simulink model "Simulink_6DoF_RV"  (R2021b)
settings: Solver=ode4  StartTime=0.0  StopTime=T_run  FixedStep=0.01  RelTol=1e-3
values from neighbouring files (symbols this model uses):
  alpha = 5    [MAIN_6DoF_RV.m]    (also in Simulatore_script_gruppo6.m)
  beta = 10    [MAIN_6DoF_RV.m]    (also in Simulatore_script_gruppo6.m)
  control = 2    [MAIN_6DoF_RV.m]    (also in Simulatore_script_gruppo6.m)
  den_pos = [Tm_pos 1]    [MAIN_6DoF_RV.m]    (also in Simulatore_script_gruppo6.m)
  dt_Fx1_PH1 = (1+dtx_PH1_corr)*dt_Fx1_PH1id    (= 48.314973357)    [MAIN_6DoF_RV.m]    (also in Simulatore_script_gruppo6.m)
  Dt_var = 0.1    [MAIN_6DoF_RV.m]    (also in Simulatore_script_gruppo6.m)
  dtz_PH2_corr = 0.28    [MAIN_6DoF_RV.m]    (also in Simulatore_script_gruppo6.m)
  epsilon = 1e-3    (= 0.001)    [MAIN_6DoF_RV.m]    (also in Simulatore_script_gruppo6.m)
  epsilon_FA = 0.005    [MAIN_6DoF_RV.m]    (also in Simulatore_script_gruppo6.m)
  F_D = 1/2*rho*CD*A*vc^2    [MAIN_6DoF_RV.m]    (also in Simulatore_script_gruppo6.m)
  fa_control = 2    [MAIN_6DoF_RV.m]    (also in Simulatore_script_gruppo6.m)
  FJ2_r4 = -mc*(3*J2*mu*r_E^2)/2    (= -1.15338103268e+24)    [MAIN_6DoF_RV.m]    (also in Simulatore_script_gruppo6.m)
  Fx_PH1id = Tmax    (= 1)    [MAIN_6DoF_RV.m]    (also in Simulatore_script_gruppo6.m)
  Fz_PH2id = Tmax    (= 1)    [MAIN_6DoF_RV.m]    (also in Simulatore_script_gruppo6.m)
  I = [Jx  0   0 ... (first row only)    [MAIN_6DoF_RV.m]    (also in Simulatore_script_gruppo6.m)
  Id = eye(3)    [MAIN_6DoF_RV.m]    (also in Simulatore_script_gruppo6.m)
  invI = inv(I)    [MAIN_6DoF_RV.m]    (also in Simulatore_script_gruppo6.m)
  K_d = diag([d1,d2,d3])    [MAIN_6DoF_RV.m]    (also in Simulatore_script_gruppo6.m)
  lambda = 0.06    [MAIN_6DoF_RV.m]    (also in Simulatore_script_gruppo6.m)
  lambda_FA = 0.07    [MAIN_6DoF_RV.m]    (also in Simulatore_script_gruppo6.m)
  mc = 43.8    [MAIN_6DoF_RV.m]    (also in Simulatore_script_gruppo6.m)
  mu = 3.986012*10^14    (= 398601200000000)    [MAIN_6DoF_RV.m]    (also in Simulatore_script_gruppo6.m)
  num_pos = Km_pos    (= 4)    [MAIN_6DoF_RV.m]    (also in Simulatore_script_gruppo6.m)
  omega = (mu/r_t^3)^0.5    (= 0.00113136572666)    [MAIN_6DoF_RV.m]    (also in Simulatore_script_gruppo6.m)
  omega_0 = [0 0 0]    [MAIN_6DoF_RV.m]    (also in Simulatore_script_gruppo6.m)
  q0_0 = 0.5    [MAIN_6DoF_RV.m]    (also in Simulatore_script_gruppo6.m)
  q0_des = quat0_PH3(1)    [MAIN_6DoF_RV.m]    (also in Simulatore_script_gruppo6.m)
  qv_0 = [0.5 0.5 0.5]    [MAIN_6DoF_RV.m]    (also in Simulatore_script_gruppo6.m)
  r0 = [Xo Yo Zo]    [MAIN_6DoF_RV.m]    (also in Simulatore_script_gruppo6.m)
  r0_p1Id = [x0_PH1, y0_PH1, z0_PH1]    [MAIN_6DoF_RV.m]    (also in Simulatore_script_gruppo6.m)
  r0_p3Id = [x0_PH3 y0_PH3 z0_PH3]    [MAIN_6DoF_RV.m]    (also in Simulatore_script_gruppo6.m)
  r_des_fa = [xf yf zf]    [MAIN_6DoF_RV.m]    (also in Simulatore_script_gruppo6.m)
  r_t = r_E + height    (= 6778145)    [MAIN_6DoF_RV.m]    (also in Simulatore_script_gruppo6.m)
  t_acc_fa = (1+dtx_PH3_corr)*t_acc_fa_id    [MAIN_6DoF_RV.m]    (also in Simulatore_script_gruppo6.m)
  tau_RW = 0.25    [MAIN_6DoF_RV.m]    (also in Simulatore_script_gruppo6.m)
  Tmax = n*Fthr    (= 1)    [MAIN_6DoF_RV.m]    (also in Simulatore_script_gruppo6.m)
  U_max = 0.25    [MAIN_6DoF_RV.m]    (also in Simulatore_script_gruppo6.m)
  U_max_RW = 1e-3    (= 0.001)    [MAIN_6DoF_RV.m]    (also in Simulatore_script_gruppo6.m)
  U_off_pos = 0.60*U_on_pos    (= 0.6)    [MAIN_6DoF_RV.m]    (also in Simulatore_script_gruppo6.m)
  U_on_pos = 1    [MAIN_6DoF_RV.m]    (also in Simulatore_script_gruppo6.m)
  v0 = [Vxo Vyo Vzo]    [MAIN_6DoF_RV.m]    (also in Simulatore_script_gruppo6.m)
  v_des_fa = [vxf vyf vzf]    [MAIN_6DoF_RV.m]    (also in Simulatore_script_gruppo6.m)
  Vx_max = 0.15    [MAIN_6DoF_RV.m]    (also in Simulatore_script_gruppo6.m)
  x0_PH2 = -3000    [MAIN_6DoF_RV.m]    (also in Simulatore_script_gruppo6.m)
  x0_PH3 = -500    [MAIN_6DoF_RV.m]    (also in Simulatore_script_gruppo6.m)
  x_start_dec = r_des_fa(1)-(v_des_fa(1)^2-(Vx_max*(1+dtx_PH3_corr))^2)/(2*(Fx_dec/mc))    [MAIN_6DoF_RV.m]    (also in Simulatore_script_gruppo6.m)
  xf = -2    [MAIN_6DoF_RV.m]    (also in Simulatore_script_gruppo6.m)
  Z0_RW = [sqrt(3)/2    0           -sqrt(3)/2  0 ... (first row only)    [MAIN_6DoF_RV.m]    (also in Simulatore_script_gruppo6.m)
  z_start_Fx2_PH1id = 0.5*(DVx2*(1+dtx_PH1_corr))^2/(Fx_PH1id/mc)    (= 26.6476786585)    [MAIN_6DoF_RV.m]    (also in Simulatore_script_gruppo6.m)
  z_start_Fz2_PH2id = 0.5*(DVz2*(1+dtz_PH2_corr))^2/(Fz_PH2id/mc)    [MAIN_6DoF_RV.m]    (also in Simulatore_script_gruppo6.m)
  Zinv = pinv(Z0_RW)    [MAIN_6DoF_RV.m]    (also in Simulatore_script_gruppo6.m)
libraries: vrlib x3, robotcorelib x1
(part 2 of 2)

== system Simulink_6DoF_RV/POSITION/Position and Guidance/Final Approach/Switch Case Action Subsystem/FA straight line ==
  Pos : Inport
  Vel : Inport  Port=2
  Action Port : ActionPort  ActionPortLabel=case [ 1 ]:
  Fx control : Subsystem
  PID y & z control : Subsystem
  Sum : Sum  Inputs=+|+
  Fc : Outport
  wires:
  PID y & z control/1(Out1) -> Sum/2
  Vel/1 -> Fx control/2(Vel), PID y & z control/2(Vel)
  Pos/1 -> PID y & z control/1(Pos), Fx control/1(Pos)
  Fx control/1(Fx) -> Sum/1
  Sum/1 -> Fc/1

== system Simulink_6DoF_RV/POSITION/Position and Guidance/Radial Boost1/ RB 2nd impulse control/Pos z y ==
  note: P=0.5 D=20 I=0
  In1 : Inport
  In2 : Inport  Port=2
  Gain : Gain  Gain=0.5
  Gain1 : Gain  Gain=0.003
  Gain2 : Gain  Gain=20
  Gain3 : Gain  Gain=[0 -1 -1]
  Gain4 : Gain  Gain=[0 -1 -1]
  Integrator : Integrator
  Sum : Sum  Inputs=+++
  Out1 : Outport
  wires:
  Gain/1 -> Sum/2
  Gain2/1 -> Sum/3
  Gain3/1 -> Integrator/1, Gain/1
  Gain1/1 -> Sum/1
  In1/1 -> Gain3/1
  Gain4/1 -> Gain2/1
  Integrator/1 -> Gain1/1
  Sum/1 -> Out1/1
  In2/1 -> Gain4/1

== system Simulink_6DoF_RV/POSITION/Position and Guidance/Radial Boost1/ RB 2nd impulse control/Vel x ==
  In1 : Inport
  Gain5 : Gain  Gain=[-1 0 0]
  Gain8 : Gain  Gain=[-10 0 0]
  Integrator1 : Integrator
  Sum1 : Sum  Inputs=|++
  Out1 : Outport
  wires:
  Gain8/1 -> Sum1/2
  Gain5/1 -> Sum1/1
  Integrator1/1 -> Gain5/1
  In1/1 -> Gain8/1, Integrator1/1
  Sum1/1 -> Out1/1

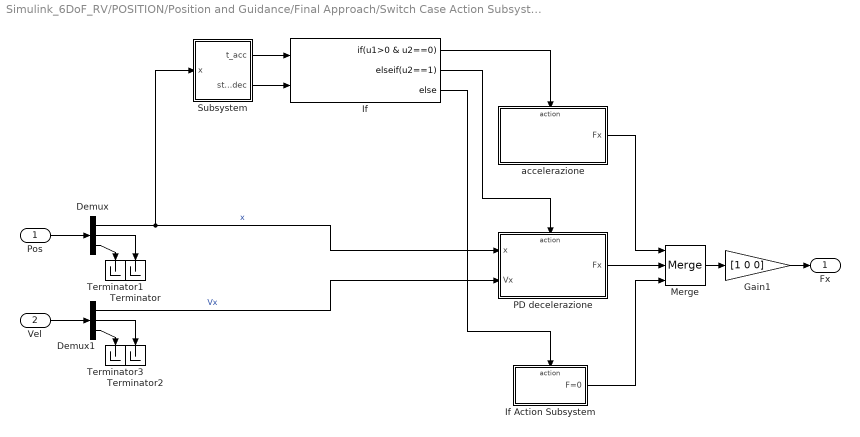
== system Simulink_6DoF_RV/POSITION/Position and Guidance/Final Approach/Switch Case Action Subsystem/FA straight line/Fx control ==
  Pos : Inport
  Vel : Inport  Port=2
  " accelerazione" : Subsystem  TreatAsAtomicUnit=on
  Demux : Demux  Outputs=3
  Demux1 : Demux  Outputs=3
  Gain1 : Gain  Gain=[1 0 0]
  If : If  NumInputs=2  IfExpression=u1>0 & u2==0  ElseIfExpressions=u2==1
  If Action Subsystem : Subsystem  TreatAsAtomicUnit=on
  Merge : Merge  Inputs=3
  PD decelerazione : Subsystem  TreatAsAtomicUnit=on
  Subsystem : Subsystem
  Terminator{,1..3} (4 alike) : Terminator
  Fx : Outport
  wires:
  Pos/1 -> Demux/1
  Demux/2 -> Terminator/1
  Demux/3 -> Terminator1/1
  " accelerazione"/1(Fx) -> Merge/1
  PD decelerazione/1(Fx) -> Merge/2
  Merge/1 -> Gain1/1
  If/2 -> PD decelerazione/Action
  If/3 -> If Action Subsystem/Action
  Demux/1 -> Subsystem/1(x), PD decelerazione/1(x)  "x"
  Gain1/1 -> Fx/1
  If Action Subsystem/1(F=0) -> Merge/3
  If/1 -> " accelerazione"/Action
  Demux1/2 -> Terminator2/1
  Vel/1 -> Demux1/1
  Demux1/3 -> Terminator3/1
  Demux1/1 -> PD decelerazione/2(Vx)  "Vx"
  Subsystem/1(t_acc) -> If/1
  Subsystem/2(start_dec) -> If/2

== system Simulink_6DoF_RV/POSITION/Position and Guidance/Final Approach/Switch Case Action Subsystem/FA straight line/PID y & z control ==
  Pos : Inport
  Vel : Inport  Port=2
  Gain : Gain  Gain=[0 -1 -1]
  Gain1 : Gain  Gain=[0 -1 -1]
  Gain4 : Gain  Gain=5
  Gain5 : Gain  Gain=0.005
  Gain6 : Gain  Gain=200
  Integrator : Integrator
  Sum : Sum  Inputs=+|+|+
  Out1 : Outport
  wires:
  Sum/1 -> Out1/1
  Vel/1 -> Gain1/1
  Pos/1 -> Gain/1
  Gain1/1 -> Gain6/1
  Gain5/1 -> Sum/1  "int"
  Gain6/1 -> Sum/3
  Gain/1 -> Integrator/1, Gain4/1
  Integrator/1 -> Gain5/1
  Gain4/1 -> Sum/2

== system Simulink_6DoF_RV/POSITION/Position and Guidance/Final Approach/Switch Case Action Subsystem/FA straight line/Fx control/ accelerazione ==
  Action Port : ActionPort  ActionPortLabel=if(u1>0 & u2==0)
  Fx_acc : Constant  Value=Tmax
  Fx : Outport
  wires:
  Fx_acc/1 -> Fx/1

== system Simulink_6DoF_RV/POSITION/Position and Guidance/Final Approach/Switch Case Action Subsystem/FA straight line/Fx control/If Action Subsystem ==
  Action Port : ActionPort  ActionPortLabel=else
  Constant : Constant  Value=0
  F=0 : Outport
  wires:
  Constant/1 -> F=0/1

== system Simulink_6DoF_RV/POSITION/Position and Guidance/Final Approach/Switch Case Action Subsystem/FA straight line/Fx control/PD decelerazione ==
  x : Inport
  Vx : Inport  Port=2
  Action Port : ActionPort  ActionPortLabel=elseif(u2==1 )
  Constant : Constant  Value=xf
  Gain : Gain  Gain=-2
  Gain1 : Gain  Gain=-0.005
  Gain2 : Gain  Gain=-50
  Integrator : Integrator
  Sum : Sum  Inputs=+++
  Sum1 : Sum  Inputs=-+|
  Fx : Outport
  wires:
  Sum1/1 -> Integrator/1, Gain/1
  Gain/1 -> Sum/2
  Gain2/1 -> Sum/3
  x/1 -> Sum1/2
  Constant/1 -> Sum1/1
  Vx/1 -> Gain2/1
  Integrator/1 -> Gain1/1
  Gain1/1 -> Sum/1
  Sum/1 -> Fx/1

== system Simulink_6DoF_RV/POSITION/Position and Guidance/Final Approach/Switch Case Action Subsystem/FA straight line/Fx control/Subsystem ==
  x : Inport
  Cast To Double2 : DataTypeConversion  OutDataTypeStr=double
  Constant : Constant  Value=x_start_dec*1.5
  Constant1 : Constant
  Constant2 : Constant  Value=t_acc_fa
  Integrator : Integrator
  Relational Operator : RelationalOperator  OutDataTypeStr=boolean  RndMeth=Simplest
  Sum : Sum  Inputs=-+|
  t_acc : Outport
  start_dec : Outport  Port=2
  wires:
  Cast To Double2/1 -> start_dec/1
  Constant1/1 -> Integrator/1
  Sum/1 -> t_acc/1
  Relational Operator/1 -> Cast To Double2/1
  Constant/1 -> Relational Operator/2
  x/1 -> Relational Operator/1
  Integrator/1 -> Sum/1
  Constant2/1 -> Sum/2

== matlab function Simulink_6DoF_RV/POSITION/Maneuvers/Subsystem3/fire-time calculator/MATLAB Function ==
  data: dt_PH2_1 output; Vel input; Pos input; data input
function dt_PH2_1 = fire_time(Vel,Pos, data)

mc=data(1);
omega=data(2);
F=data(3);
X_fin=data(4);
dt_corr=data(5);
dX=X_fin-Pos(1);
Vz_fin=omega*dX/4;
DV=Vz_fin-Vel(3);
dt_PH2_1 = DV*mc/F*(1+dt_corr);
end

== matlab function Simulink_6DoF_RV/ATTITUDE/SMC/MATLAB Function ==
  data: omega_B input; y output; qv input; max input; ctrl_var input; control input
function y  = SMC(omega_B,qv,max,ctrl_var,control)

lambda = ctrl_var(1);   %0.5 funiona bene
epsilon = ctrl_var(2);
if control==1
K = max(1);
else
K = max(2);
end

sigma = (omega_B+lambda*(qv));

%     if (abs(sigma) > epsilon)    
%         sigma1=sign(sigma);
%     else
%         sigma1=sigma/epsilon;
% 
%     end
sigma1=tanh(sigma/epsilon);

y= -K*sigma1;
end

== matlab function Simulink_6DoF_RV/POSITION/Position and Guidance/Final Approach/Switch Case Action Subsystem/FA SMC/MATLAB Function ==
  data: Vel input; F output; Pos input; max input; ctrl_var input; Vx_max input; omega_mc input
function F = SMC(Vel,Pos,max,ctrl_var,Vx_max,omega_mc)

lambda = ctrl_var(1);  
epsilon = ctrl_var(2);
K=max;

sigma = (Vel+lambda*(Pos));
sigma1=zeros(3,1);
for i=1:length(sigma)
    if (abs(sigma(i)) > epsilon)    
        sigma1(i)=sign(sigma(i));
    else
        sigma1(i)=sigma(i)/epsilon;
    end     
end

F= -K*sigma1;

if Vel(1)>=Vx_max && F(1)>0
    F=-K*[0 sigma1(2) sigma1(3)]';
elseif  Vel(1)<=-Vx_max && F(1)<0
    F=-K*[0 sigma1(2) sigma1(3)]';
end

F(3)=F(3)+3*omega_mc(1)^2*Pos(3)*omega_mc(2)-2*omega_mc(1)*Vel(1)*omega_mc(2);

end
